simulink model "simulation"  (R2016a)
settings: Solver=ode45  StartTime=0.0  StopTime=30  FixedStep=0.01  MaxStep=0.01  RelTol=1e-3
values from neighbouring files (symbols this model uses):
  f_thrust_limit_up = m*g+z_dot_limit_up^2*k_aer_z*m    (= 5.2245)    [main.m]
  g = 9.81    [main.m]
  k_aer_x = 0.1    [main.m]
  k_aer_y = 0.1    [main.m]
  k_aer_z = 0.2    [main.m]
  kdp = 15    [main.m]
  kdps = 15    [main.m]
  kdt = 15    [main.m]
  kdx = 1    [main.m]
  kdy = 1    [main.m]
  kdz = 20    [main.m]
  kpp = 100    [main.m]
  kpps = 100    [main.m]
  kpt = 100    [main.m]
  kpx = 1.2    [main.m]
  kpy = 1.2    [main.m]
  kpz = 100    [main.m]
  m = 0.45    [main.m]
  max_phi = 0.05    [main.m]
  max_theta = 0.05    [main.m]
settings Model: Creator=Jens  LastModifiedBy=Jens

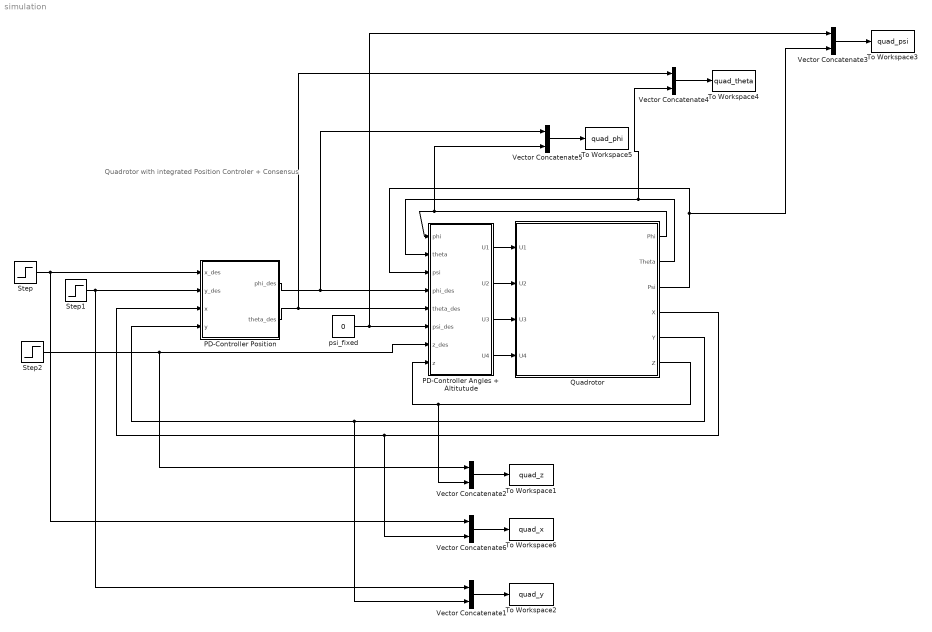
== system simulation ==
  note: Quadrotor with integrated Position Controler
      | + Consensus
  PD-Controller Angles + Altitutude : Subsystem
  PD-Controller Position : Subsystem
  Quadrotor : Subsystem
  Step : Step  Time=2  After=30  SampleTime=0
  Step1 : Step  Time=2  After=0  SampleTime=0
  Step2 : Step  Time=2  After=0  SampleTime=0
  To Workspace1 : ToWorkspace  VariableName=quad_z  SaveFormat=Timeseries  SampleTime=-1
  To Workspace2 : ToWorkspace  VariableName=quad_y  SaveFormat=Timeseries  SampleTime=-1
  To Workspace3 : ToWorkspace  VariableName=quad_psi  SaveFormat=Timeseries  SampleTime=-1
  To Workspace4 : ToWorkspace  VariableName=quad_theta  SaveFormat=Timeseries  SampleTime=-1
  To Workspace5 : ToWorkspace  VariableName=quad_phi  SaveFormat=Timeseries  SampleTime=-1
  To Workspace6 : ToWorkspace  VariableName=quad_x  SaveFormat=Timeseries  SampleTime=-1
  Vector Concatenate{1..6} (6 alike) : Concatenate
  psi_fixed : Constant  Value=0
  wires:
  Quadrotor/6(Z) -> Vector Concatenate2/2, PD-Controller Angles + Altitutude/8(z)
  Quadrotor/5(Y) -> Vector Concatenate1/2, PD-Controller Position/4(y)
  Quadrotor/4(X) -> Vector Concatenate6/2, PD-Controller Position/3(x)
  psi_fixed/1 -> Vector Concatenate3/1, PD-Controller Angles + Altitutude/6(psi_des)
  Step/1 -> Vector Concatenate6/1, PD-Controller Position/1(x_des)
  Step1/1 -> Vector Concatenate1/1, PD-Controller Position/2(y_des)
  PD-Controller Angles + Altitutude/4(U4) -> Quadrotor/4(U4)
  PD-Controller Angles + Altitutude/2(U2) -> Quadrotor/2(U2)
  PD-Controller Angles + Altitutude/3(U3) -> Quadrotor/3(U3)
  Quadrotor/1(Phi) -> Vector Concatenate5/2, PD-Controller Angles + Altitutude/1(phi)
  Step2/1 -> Vector Concatenate2/1, PD-Controller Angles + Altitutude/7(z_des)
  PD-Controller Position/2(theta_des) -> Vector Concatenate4/1, PD-Controller Angles + Altitutude/5(theta_des)
  Quadrotor/2(Theta) -> Vector Concatenate4/2, PD-Controller Angles + Altitutude/2(theta)
  PD-Controller Position/1(phi_des) -> Vector Concatenate5/1, PD-Controller Angles + Altitutude/4(phi_des)
  Quadrotor/3(Psi) -> Vector Concatenate3/2, PD-Controller Angles + Altitutude/3(psi)
  PD-Controller Angles + Altitutude/1(U1) -> Quadrotor/1(U1)
  Vector Concatenate2/1 -> To Workspace1/1
  Vector Concatenate1/1 -> To Workspace2/1
  Vector Concatenate3/1 -> To Workspace3/1
  Vector Concatenate4/1 -> To Workspace4/1
  Vector Concatenate5/1 -> To Workspace5/1
  Vector Concatenate6/1 -> To Workspace6/1

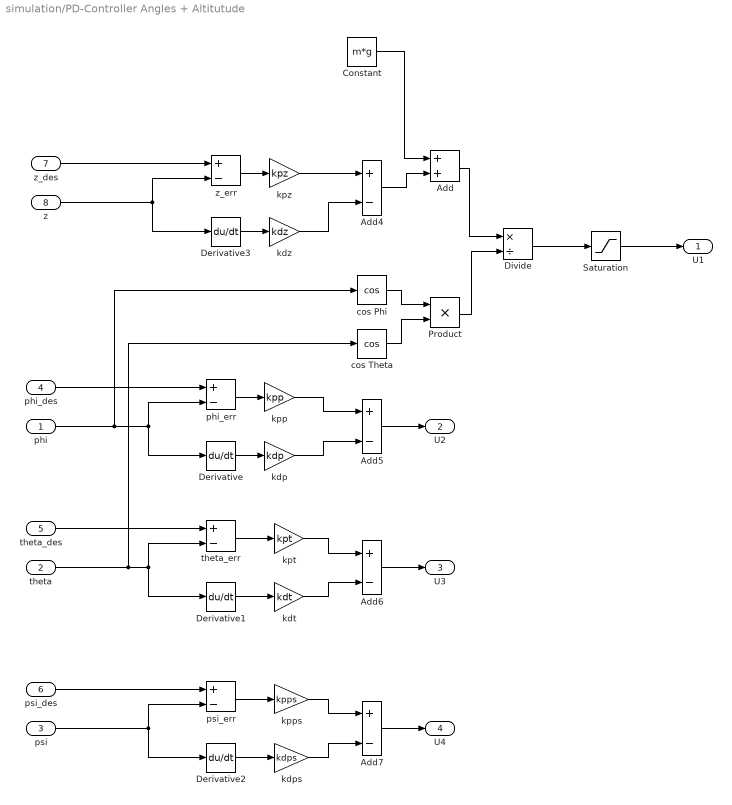
== system simulation/PD-Controller Angles + Altitutude ==
  phi : Inport
  theta : Inport  Port=2
  psi : Inport  Port=3
  phi_des : Inport  Port=4
  theta_des : Inport  Port=5
  psi_des : Inport  Port=6
  z_des : Inport  Port=7
  z : Inport  Port=8
  Add : Sum
  Add{4..7} (4 alike) : Sum  Inputs=+-
  Constant : Constant  Value=m*g
  Derivative{,1..3} (4 alike) : Derivative
  Divide : Product  Inputs=*/
  Product : Product  RndMeth=Zero
  Saturation : Saturate  UpperLimit=f_thrust_limit_up  LowerLimit=0  ZeroCross=off
  cos Phi : Trigonometry  Operator=cos
  cos Theta : Trigonometry  Operator=cos
  kdp : Gain  Gain=kdp
  kdps : Gain  Gain=kdps
  kdt : Gain  Gain=kdt
  kdz : Gain  Gain=kdz
  kpp : Gain  Gain=kpp
  kpps : Gain  Gain=kpps
  kpt : Gain  Gain=kpt
  kpz : Gain  Gain=kpz
  phi_err : Sum  Inputs=+-
  psi_err : Sum  Inputs=+-
  theta_err : Sum  Inputs=+-
  z_err : Sum  Inputs=+-
  U1 : Outport
  U2 : Outport  Port=2
  U3 : Outport  Port=3
  U4 : Outport  Port=4
  wires:
  phi/1 -> Derivative/1, phi_err/2, cos Phi/1
  theta/1 -> Derivative1/1, theta_err/2, cos Theta/1
  psi/1 -> Derivative2/1, psi_err/2
  phi_des/1 -> phi_err/1
  theta_des/1 -> theta_err/1
  psi_des/1 -> psi_err/1
  phi_err/1 -> kpp/1
  Derivative/1 -> kdp/1
  theta_err/1 -> kpt/1
  Derivative1/1 -> kdt/1
  psi_err/1 -> kpps/1
  Derivative2/1 -> kdps/1
  z/1 -> Derivative3/1, z_err/2
  z_des/1 -> z_err/1
  z_err/1 -> kpz/1
  Derivative3/1 -> kdz/1
  kpz/1 -> Add4/1
  kdz/1 -> Add4/2
  kpp/1 -> Add5/1
  kdp/1 -> Add5/2
  Add5/1 -> U2/1
  kpt/1 -> Add6/1
  kdt/1 -> Add6/2
  Add6/1 -> U3/1
  kpps/1 -> Add7/1
  kdps/1 -> Add7/2
  Add7/1 -> U4/1
  cos Phi/1 -> Product/1
  cos Theta/1 -> Product/2
  Add4/1 -> Add/2
  Add/1 -> Divide/1
  Product/1 -> Divide/2
  Constant/1 -> Add/1
  Saturation/1 -> U1/1
  Divide/1 -> Saturation/1

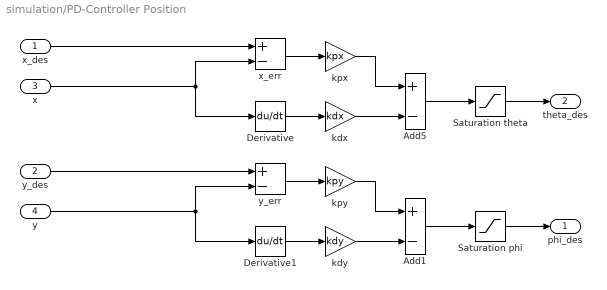
== system simulation/PD-Controller Position ==
  x_des : Inport
  y_des : Inport  Port=2
  x : Inport  Port=3
  y : Inport  Port=4
  Add1 : Sum  Inputs=+-
  Add5 : Sum  Inputs=+-
  Derivative : Derivative
  Derivative1 : Derivative
  Saturation phi : Saturate  UpperLimit=max_phi  LowerLimit=-max_phi  ZeroCross=off
  Saturation theta : Saturate  UpperLimit=max_theta  LowerLimit=-max_theta  ZeroCross=off
  kdx : Gain  Gain=kdx
  kdy : Gain  Gain=kdy
  kpx : Gain  Gain=kpx
  kpy : Gain  Gain=kpy
  x_err : Sum  Inputs=+-
  y_err : Sum  Inputs=+-
  phi_des : Outport
  theta_des : Outport  Port=2
  wires:
  x/1 -> Derivative/1, x_err/2
  x_des/1 -> x_err/1
  x_err/1 -> kpx/1
  Derivative/1 -> kdx/1
  kpx/1 -> Add5/1
  kdx/1 -> Add5/2
  Add5/1 -> Saturation theta/1
  y/1 -> Derivative1/1, y_err/2
  y_err/1 -> kpy/1
  Derivative1/1 -> kdy/1
  kpy/1 -> Add1/1
  Add1/1 -> Saturation phi/1
  y_des/1 -> y_err/1
  Saturation theta/1 -> theta_des/1
  Saturation phi/1 -> phi_des/1
  kdy/1 -> Add1/2

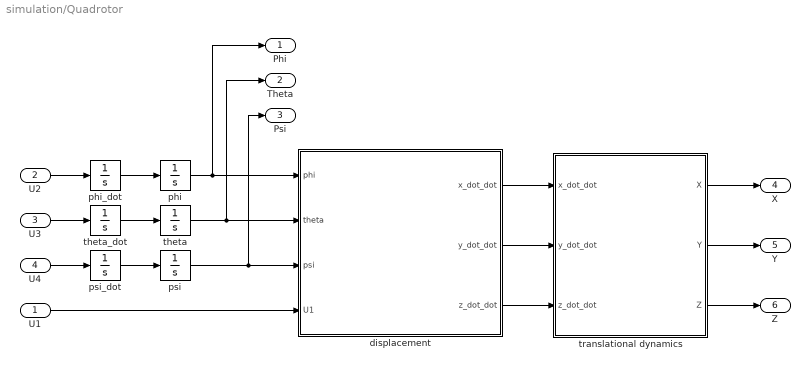
== system simulation/Quadrotor ==
  U1 : Inport
  U2 : Inport  Port=2
  U3 : Inport  Port=3
  U4 : Inport  Port=4
  displacement : Subsystem
  phi : Integrator  ZeroCross=off
  phi_dot : Integrator
  psi : Integrator  ZeroCross=off
  psi_dot : Integrator  ZeroCross=off
  theta : Integrator  ZeroCross=off
  theta_dot : Integrator  ZeroCross=off
  translational dynamics : Subsystem
  Phi : Outport
  Theta : Outport  Port=2
  Psi : Outport  Port=3
  X : Outport  Port=4
  Y : Outport  Port=5
  Z : Outport  Port=6
  wires:
  U2/1 -> phi_dot/1
  U3/1 -> theta_dot/1
  U4/1 -> psi_dot/1
  phi_dot/1 -> phi/1
  theta_dot/1 -> theta/1
  psi_dot/1 -> psi/1
  phi/1 -> displacement/1(phi), Phi/1
  theta/1 -> displacement/2(theta), Theta/1
  psi/1 -> Psi/1, displacement/3(psi)
  U1/1 -> displacement/4(U1)
  displacement/1(x_dot_dot) -> translational dynamics/1(x_dot_dot)
  displacement/2(y_dot_dot) -> translational dynamics/2(y_dot_dot)
  displacement/3(z_dot_dot) -> translational dynamics/3(z_dot_dot)
  translational dynamics/1(X) -> X/1
  translational dynamics/2(Y) -> Y/1
  translational dynamics/3(Z) -> Z/1

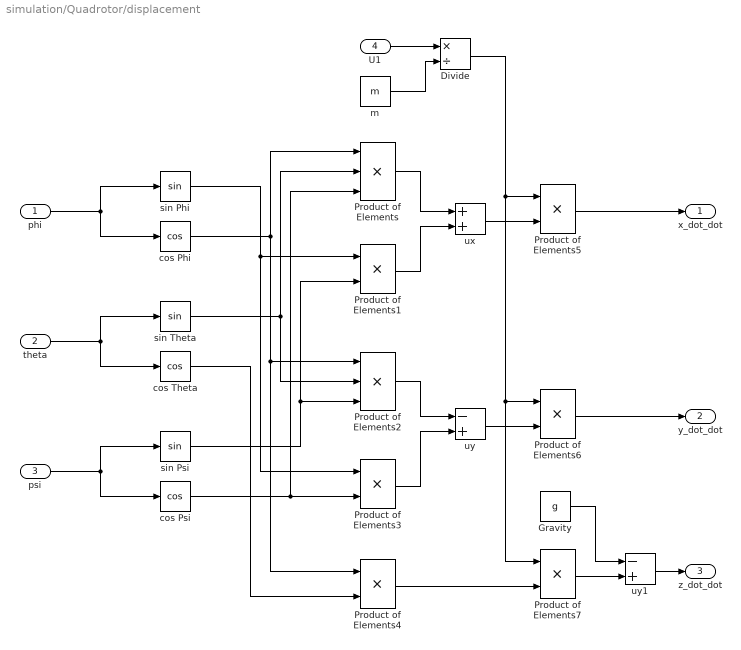
== system simulation/Quadrotor/displacement ==
  phi : Inport
  theta : Inport  Port=2
  psi : Inport  Port=3
  U1 : Inport  Port=4
  Divide : Product  Inputs=*/
  Gravity : Constant  Value=g
  Product of Elements : Product  Inputs=3
  Product of Elements{1,3..7} (6 alike) : Product
  Product of Elements2 : Product  Inputs=3
  cos Phi : Trigonometry  Operator=cos
  cos Psi : Trigonometry  Operator=cos
  cos Theta : Trigonometry  Operator=cos
  m : Constant  Value=m
  sin Phi : Trigonometry
  sin Psi : Trigonometry
  sin Theta : Trigonometry
  ux : Sum
  uy : Sum  Inputs=-+
  uy1 : Sum  Inputs=-+
  x_dot_dot : Outport
  y_dot_dot : Outport  Port=2
  z_dot_dot : Outport  Port=3
  wires:
  phi/1 -> sin Phi/1, cos Phi/1
  theta/1 -> sin Theta/1, cos Theta/1
  psi/1 -> sin Psi/1, cos Psi/1
  sin Theta/1 -> Product of Elements/2, Product of Elements2/2
  cos Psi/1 -> Product of Elements/3, Product of Elements3/2
  cos Phi/1 -> Product of Elements/1, Product of Elements2/1, Product of Elements4/1
  sin Phi/1 -> Product of Elements1/1, Product of Elements3/1
  sin Psi/1 -> Product of Elements1/2, Product of Elements2/3
  Product of Elements/1 -> ux/1
  Product of Elements1/1 -> ux/2
  ux/1 -> Product of Elements5/2
  Product of Elements2/1 -> uy/1
  Product of Elements3/1 -> uy/2
  uy/1 -> Product of Elements6/2
  cos Theta/1 -> Product of Elements4/2
  Product of Elements4/1 -> Product of Elements7/2
  U1/1 -> Divide/1
  m/1 -> Divide/2
  Divide/1 -> Product of Elements5/1, Product of Elements6/1, Product of Elements7/1
  Product of Elements5/1 -> x_dot_dot/1
  Product of Elements6/1 -> y_dot_dot/1
  uy1/1 -> z_dot_dot/1
  Product of Elements7/1 -> uy1/2
  Gravity/1 -> uy1/1

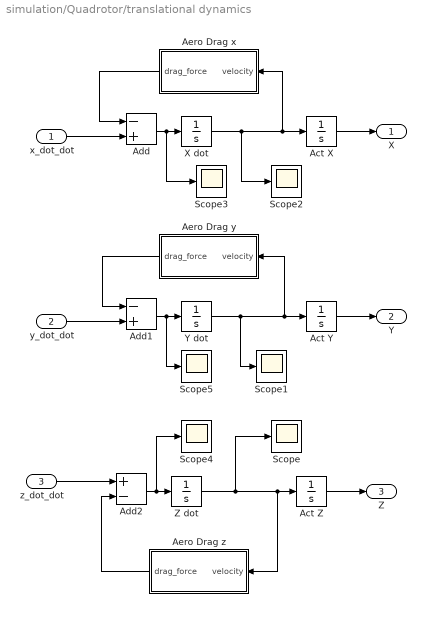
== system simulation/Quadrotor/translational dynamics ==
  x_dot_dot : Inport
  y_dot_dot : Inport  Port=2
  z_dot_dot : Inport  Port=3
  Act X : Integrator
  Act Y : Integrator
  Act Z : Integrator
  Add : Sum  Inputs=-+
  Add1 : Sum  Inputs=-+
  Add2 : Sum  Inputs=+-
  Aero Drag x : Subsystem
  Aero Drag y : Subsystem
  Aero Drag z : Subsystem
  Scope{,1..5} (6 alike) : Scope
  X dot : Integrator
  Y dot : Integrator
  Z dot : Integrator
  X : Outport
  Y : Outport  Port=2
  Z : Outport  Port=3
  wires:
  Add1/1 -> Scope5/1, Y dot/1
  Act Z/1 -> Z/1
  X dot/1 -> Scope2/1, Act X/1, Aero Drag x/1(velocity)
  Act Y/1 -> Y/1
  Aero Drag x/1(drag_force) -> Add/1
  y_dot_dot/1 -> Add1/2
  Y dot/1 -> Scope1/1, Aero Drag y/1(velocity), Act Y/1
  Aero Drag z/1(drag_force) -> Add2/2
  x_dot_dot/1 -> Add/2
  Aero Drag y/1(drag_force) -> Add1/1
  Z dot/1 -> Scope/1, Aero Drag z/1(velocity), Act Z/1
  Act X/1 -> X/1
  Add2/1 -> Scope4/1, Z dot/1
  z_dot_dot/1 -> Add2/1
  Add/1 -> Scope3/1, X dot/1

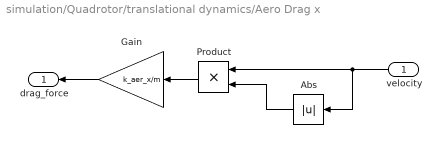
== system simulation/Quadrotor/translational dynamics/Aero Drag x ==
  velocity : Inport
  Abs : Abs
  Gain : Gain  Gain=k_aer_x/m
  Product : Product
  drag_force : Outport
  wires:
  Product/1 -> Gain/1
  velocity/1 -> Product/1, Abs/1
  Gain/1 -> drag_force/1
  Abs/1 -> Product/2

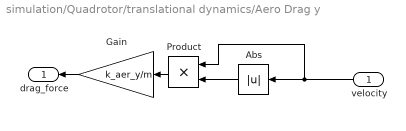
== system simulation/Quadrotor/translational dynamics/Aero Drag y ==
  velocity : Inport
  Abs : Abs
  Gain : Gain  Gain=k_aer_y/m
  Product : Product
  drag_force : Outport
  wires:
  Product/1 -> Gain/1
  velocity/1 -> Product/1, Abs/1
  Gain/1 -> drag_force/1
  Abs/1 -> Product/2

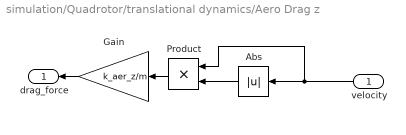
== system simulation/Quadrotor/translational dynamics/Aero Drag z ==
  velocity : Inport
  Abs : Abs
  Gain : Gain  Gain=k_aer_z/m
  Product : Product
  drag_force : Outport
  wires:
  Product/1 -> Gain/1
  velocity/1 -> Product/1, Abs/1
  Gain/1 -> drag_force/1
  Abs/1 -> Product/2
